simulink model "PI_controller"  (R2019a)
settings: Solver=VariableStepAuto  StartTime=0.0  StopTime=100  RelTol=1e-3
values from neighbouring files (symbols this model uses):
  g = 9.81    [Data.m]    (also in func.m; myTransitionFcn.m)
  m = 0.1    [Data.m]    (also in myTransitionFcn.m)
  r = 0.1    [Data.m]    (also in func.m; myTransitionFcn.m)
  R = 1    [Data.m]    (also in func.m; myTransitionFcn.m)
libraries: simulink x1
settings Model: Creator=Dell  LastModifiedBy=Dell

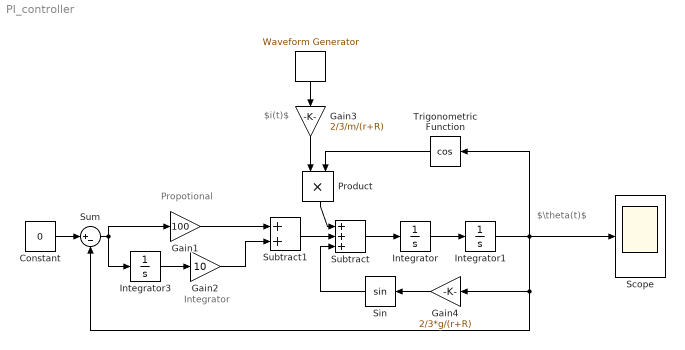
== system PI_controller ==
  note: Integrator
  note: Propotional
  note: $i(t)$
  note: $\theta(t)$
  " " : simulink/Sources/Waveform Generator  OutMin=[]  OutMax=[]  OutDataTypeStr=double  SelectedSignal=1  Signals=step()  BlockNames=MultiportSwitch_8c7b78d12e5b405  SampleTime=0.1
      settings: SourceProductName=Simulink
  Constant : Constant  Value=0
  Gain1 : Gain  Gain=100
  Gain2 : Gain  Gain=10
  Gain3 : Gain  Gain=2/3/m/(r+R)
  Gain4 : Gain  Gain=2/3*g/(r+R)
  Integrator : Integrator
  Integrator1 : Integrator
  Integrator3 : Integrator
  Product : Product
  Scope : Scope
  Sin : Trigonometry
  Subtract : Sum  Inputs=+++
  Subtract1 : Sum
  Sum : Sum  Inputs=|+-
  Trigonometric Function : Trigonometry  Operator=cos
  wires:
  Gain3/1 -> Product/1
  Integrator1/1 -> Scope/1, Trigonometric Function/1, Gain4/1, Sum/2
  Integrator/1 -> Integrator1/1
  Trigonometric Function/1 -> Product/2
  Constant/1 -> Sum/1
  Sin/1 -> Subtract/3
  Sum/1 -> Gain1/1, Integrator3/1
  Gain4/1 -> Sin/1
  Subtract/1 -> Integrator/1
  Product/1 -> Subtract/1
  " "/1 -> Gain3/1
  Subtract1/1 -> Subtract/2
  Integrator3/1 -> Gain2/1
  Gain1/1 -> Subtract1/1
  Gain2/1 -> Subtract1/2
